simulink model "iddemo_engine"  (R2016a)
settings: Solver=ode45  StartTime=0.0  StopTime=200  MaxStep=0.01  RelTol=1e-3
model workspace (MAT data in the model file):
  Adist = -0.7
  N = 2000
  Tdist = 200
  Ts = 0.003
  p = [-7.82997288351e-05; 0.181210895977; -0.072497134344; 0.000486358314052; 0.0361674637937]
undefined symbols (not defined in the file or in its folder): magnitude
libraries: simulink x1, slident x1
settings Model: Creator=The MathWorks, Inc.  LastModifiedBy=The MathWorks, Inc.
settings DataIOCC: LimitDataPoints=on  SaveFormat=Array
settings DebuggingCC: SolverPrmCheckMsg=warning
settings HardwareCC: ProdBitPerPointer=32  ProdLargestAtomicFloat=None  ProdIntDivRoundTo=Undefined  ProdEndianess=Unspecified  ProdWordSize=32  ProdHWDeviceType=32-bit Generic
settings ModelReferenceCC: PropagateSignalLabelsOutOfModel=off
settings SFSimCC: SimGenImportedTypeDefs=on
settings ConfigComp: CovModelRefEnable=Off  CovSFcnEnable=off

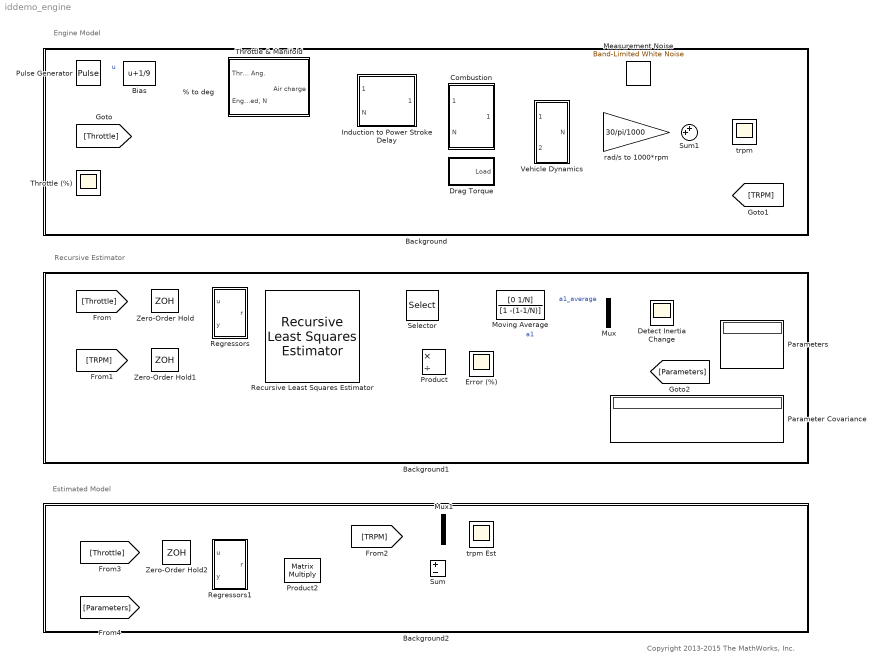
== system iddemo_engine ==
  note: Copyright 2013-2015 The MathWorks, Inc.
  note: Engine Model
  note: Recursive Estimator
  note: Estimated Model
  "% to deg " : Gain  Gain=90  SaturateOnIntegerOverflow=on  OutDataTypeStr=Inherit: Same as input  ParamDataTypeStr=Inherit: Same as input
  Background : Subsystem
      mask Display: disp('')
  Background1 : Subsystem
      mask Display: disp('')
  Background2 : Subsystem
      mask Display: disp('')
  Bias : Bias  Bias=1/9
  Combustion : Subsystem
      settings: RTWMemSecFuncInitTerm=Default  RTWMemSecFuncExecute=Default  RTWMemSecDataConstants=Default  RTWMemSecDataInternal=Default  RTWMemSecDataParameters=Default
  Detect Inertia Change : Scope
  Drag Torque : Subsystem
      settings: RTWMemSecFuncInitTerm=Default  RTWMemSecFuncExecute=Default  RTWMemSecDataConstants=Default  RTWMemSecDataInternal=Default  RTWMemSecDataParameters=Default
  Error (%) : Scope
  Induction to Power Stroke Delay : Subsystem
      settings: RTWMemSecFuncInitTerm=Default  RTWMemSecFuncExecute=Default  RTWMemSecDataConstants=Default  RTWMemSecDataInternal=Default  RTWMemSecDataParameters=Default
  Measurement Noise : simulink/Sources/Band-Limited White Noise  Cov=1e-5  Ts=Ts  seed=[23341]
  Moving Average : DiscreteFilter  Numerator=[0 1/N]  Denominator=[1 -(1-1/N)]
  Mux : Mux  Inputs=2
  Mux1 : Mux  Inputs=2
  Parameter Covariance : Display
  Parameters : Display
  Product : Product  Inputs=*/
  Product2 : Product  Multiplication=Matrix(*)
  Pulse Generator : DiscretePulseGenerator  PulseType=Time based  Amplitude=7/9  Period=20  PulseWidth=50
  Recursive Least Squares Estimator : slident/Estimators/Recursive Least Squares Estimator  InitialEstimateSource=None  InitialParameterData=3  P0=1  EstimationMethod=Forgetting Factor  AdaptationParameter=1-2e-4  NormalizationBias=eps  OutputError=on  OutputP=on  AddEnablePort=off  Ts=Ts
  Regressors : Subsystem
  Regressors1 : Subsystem
  Selector : Selector  InputPortWidth=3  IndexOptions=Index vector (dialog)  Indices=1  OutputSizes=1
  Sum : Sum  Inputs=+-
  Sum1 : Sum  Inputs=++|
  Throttle & Manifold : Subsystem
      settings: RTWMemSecFuncInitTerm=Default  RTWMemSecFuncExecute=Default  RTWMemSecDataConstants=Default  RTWMemSecDataInternal=Default  RTWMemSecDataParameters=Default
  Throttle (%) : Scope
  Vehicle Dynamics : Subsystem
      settings: RTWMemSecFuncInitTerm=Default  RTWMemSecFuncExecute=Default  RTWMemSecDataConstants=Default  RTWMemSecDataInternal=Default  RTWMemSecDataParameters=Default
  Zero-Order Hold : ZeroOrderHold  SampleTime=Ts
  Zero-Order Hold1 : ZeroOrderHold  SampleTime=Ts
  Zero-Order Hold2 : ZeroOrderHold  SampleTime=Ts
  rad/s to 1000*rpm : Gain  Gain=30/pi/1000  SaturateOnIntegerOverflow=on  OutDataTypeStr=Inherit: Same as input  ParamDataTypeStr=Inherit: Same as input
  trpm : Scope
  trpm Est : Scope  NumInputPorts=2
  wires:
  Throttle & Manifold/1(Air charge) -> Induction to Power Stroke Delay/1(Air charge)
  Vehicle Dynamics/1(N) -> Combustion/2(N), Induction to Power Stroke Delay/2(N), Throttle & Manifold/2("Engine Speed, N"), rad/s to 1000*rpm/1
  Combustion/1(Torque) -> Vehicle Dynamics/1(Teng)
  Drag Torque/1(Load) -> Vehicle Dynamics/2(Tload)
  Induction to Power Stroke Delay/1(Air Charge) -> Combustion/1(Air Charge)
  Pulse Generator/1 -> Bias/1  "u"
  Bias/1 -> Throttle (%)/1, [Throttle], "% to deg "/1
  Regressors/1(r) -> Recursive Least Squares Estimator/1
  Recursive Least Squares Estimator/1 -> Selector/1, [Parameters], Parameters/1
  Recursive Least Squares Estimator/2 -> Product/1
  Product/1 -> Error (%)/1
  [TRPM] -> Zero-Order Hold1/1
  Recursive Least Squares Estimator/3 -> Parameter Covariance/1
  Selector/1 -> Mux/2, Moving Average/1  "a1"
  [Throttle] -> Zero-Order Hold/1
  Moving Average/1 -> Mux/1  "a1_average"
  Mux/1 -> Detect Inertia Change/1
  Sum/1 -> trpm Est/2
  Regressors1/1(r) -> Product2/1
  [Throttle] -> Zero-Order Hold2/1
  [TRPM] -> Sum/1, Mux1/2
  Mux1/1 -> trpm Est/1
  Sum1/1 -> [TRPM], trpm/1
  rad/s to 1000*rpm/1 -> Sum1/2
  Measurement Noise/1 -> Sum1/1
  Zero-Order Hold/1 -> Regressors/1(u)
  Zero-Order Hold1/1 -> Recursive Least Squares Estimator/2, Regressors/2(y), Product/2
  Zero-Order Hold2/1 -> Regressors1/1(u)
  Product2/1 -> Sum/2, Regressors1/2(y), Mux1/1
  [Parameters] -> Product2/2
  "% to deg "/1 -> Throttle & Manifold/1(Throttle Ang.)

== system iddemo_engine/Background ==

== system iddemo_engine/Background1 ==

== system iddemo_engine/Background2 ==

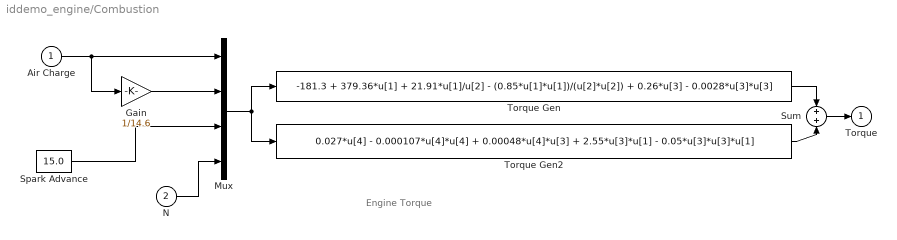
== system iddemo_engine/Combustion ==
  note: Engine Torque
  Air Charge : Inport
  N : Inport  Port=2
  Gain : Gain  Gain=1/14.6
  Mux : Mux
  Spark Advance : Constant  Value=15.0
  Sum : Sum  SaturateOnIntegerOverflow=on  InputSameDT=on  OutDataTypeStr=Inherit: Same as first input
  Torque Gen : Fcn  Expr=-181.3 + 379.36*u[1] + 21.91*u[1]/u[2] - (0.85*u[1]*u[1])/(u[2]*u[2]) + 0.26*u[3] - 0.0028*u[3]*u[3]
  Torque Gen2 : Fcn  Expr=0.027*u[4] - 0.000107*u[4]*u[4] + 0.00048*u[4]*u[3] + 2.55*u[3]*u[1] - 0.05*u[3]*u[3]*u[1]
  Torque : Outport  InitialOutput=0
  wires:
  Spark Advance/1 -> Mux/3
  N/1 -> Mux/4
  Air Charge/1 -> Gain/1, Mux/1
  Mux/1 -> Torque Gen/1, Torque Gen2/1
  Torque Gen2/1 -> Sum/2
  Torque Gen/1 -> Sum/1
  Sum/1 -> Torque/1
  Gain/1 -> Mux/2

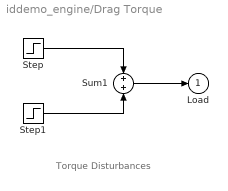
== system iddemo_engine/Drag Torque ==
  note: Torque Disturbances
  Step : Step  Time=45  After=0  SampleTime=0
  Step1 : Step  Time=45  After=0  SampleTime=0
  Sum1 : Sum  SaturateOnIntegerOverflow=on  InputSameDT=on  OutDataTypeStr=Inherit: Same as first input
  Load : Outport  InitialOutput=0
  wires:
  Step1/1 -> Sum1/2
  Step/1 -> Sum1/1
  Sum1/1 -> Load/1

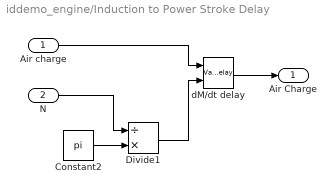
== system iddemo_engine/Induction to Power Stroke Delay ==
  Air charge : Inport
  N : Inport  Port=2
  Constant2 : Constant  Value=pi
  Divide1 : Product  Inputs=/*
  dM/dt delay : VariableTransportDelay  MaximumDelay=10  InitialOutput=0.152231307101552  MaximumPoints=5120  TransDelayFeedthrough=on  PadeOrder=2
  Air Charge : Outport
  wires:
  dM/dt delay/1 -> Air Charge/1
  Constant2/1 -> Divide1/2
  N/1 -> Divide1/1
  Divide1/1 -> dM/dt delay/2
  Air charge/1 -> dM/dt delay/1

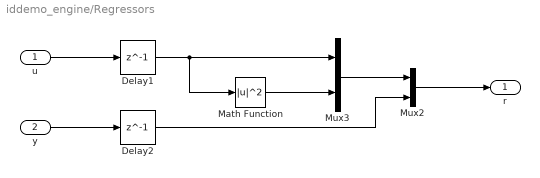
== system iddemo_engine/Regressors ==
  u : Inport
  y : Inport  Port=2
  Delay1 : Delay  DelayLength=1  InitialCondition=1  SampleTime=Ts
  Delay2 : Delay  DelayLength=1  InitialCondition=2  SampleTime=Ts
  Math Function : Math  Operator=magnitude^2  SaturateOnIntegerOverflow=on
  Mux2 : Mux  Inputs=2
  Mux3 : Mux  Inputs=2
  r : Outport
  wires:
  u/1 -> Delay1/1
  Mux2/1 -> r/1
  Delay1/1 -> Math Function/1, Mux3/1
  y/1 -> Delay2/1
  Mux3/1 -> Mux2/1
  Delay2/1 -> Mux2/2
  Math Function/1 -> Mux3/2

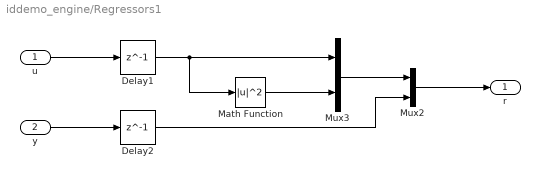
== system iddemo_engine/Regressors1 ==
  u : Inport
  y : Inport  Port=2
  Delay1 : Delay  DelayLength=1  InitialCondition=1  SampleTime=Ts
  Delay2 : Delay  DelayLength=1  InitialCondition=2  SampleTime=Ts
  Math Function : Math  Operator=magnitude^2  SaturateOnIntegerOverflow=on
  Mux2 : Mux  Inputs=2
  Mux3 : Mux  Inputs=2
  r : Outport
  wires:
  u/1 -> Delay1/1
  Mux2/1 -> r/1
  Delay1/1 -> Math Function/1, Mux3/1
  y/1 -> Delay2/1
  Mux3/1 -> Mux2/1
  Delay2/1 -> Mux2/2
  Math Function/1 -> Mux3/2

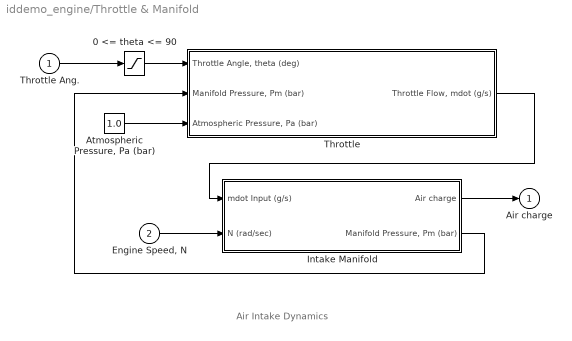
== system iddemo_engine/Throttle & Manifold ==
  note: Air Intake Dynamics
  Throttle Ang. : Inport
  "Engine Speed, N" : Inport  Port=2
  0 <= theta <= 90 : Saturate  UpperLimit=90  LowerLimit=0
  "Atmospheric Pressure, Pa (bar)" : Constant  Value=1.0
  Intake Manifold : Subsystem
      settings: RTWMemSecFuncInitTerm=Default  RTWMemSecFuncExecute=Default  RTWMemSecDataConstants=Default  RTWMemSecDataInternal=Default  RTWMemSecDataParameters=Default
  Throttle : Subsystem
      settings: RTWMemSecFuncInitTerm=Default  RTWMemSecFuncExecute=Default  RTWMemSecDataConstants=Default  RTWMemSecDataInternal=Default  RTWMemSecDataParameters=Default
  Air charge : Outport  InitialOutput=0
  wires:
  Intake Manifold/1(Air charge) -> Air charge/1
  Intake Manifold/2("Manifold Pressure, Pm (bar)") -> Throttle/2("Manifold Pressure, Pm (bar)")
  "Engine Speed, N"/1 -> Intake Manifold/2(N (rad/sec))
  Throttle/1("Throttle Flow, mdot (g/s)") -> Intake Manifold/1(mdot Input (g/s))
  Throttle Ang./1 -> 0 <= theta <= 90/1
  0 <= theta <= 90/1 -> Throttle/1("Throttle Angle, theta (deg)")
  "Atmospheric Pressure, Pa (bar)"/1 -> Throttle/3("Atmospheric Pressure, Pa (bar) ")

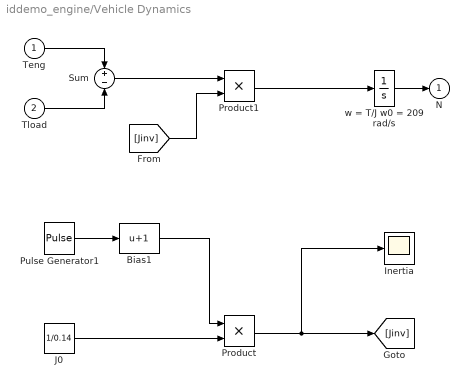
== system iddemo_engine/Vehicle Dynamics ==
  Teng : Inport
  Tload : Inport  Port=2
  Bias1 : Bias  Bias=1
  Inertia : Scope
  J0 : Constant  Value=1/0.14
  Product : Product
  Product1 : Product
  Pulse Generator1 : DiscretePulseGenerator  PulseType=Time based  Amplitude=Adist  Period=Tdist  PulseWidth=50  PhaseDelay=Tdist/2
  Sum : Sum  Inputs=+-  SaturateOnIntegerOverflow=on  InputSameDT=on  OutDataTypeStr=Inherit: Same as first input
  w = T/J w0 = 209 rad/s : Integrator  InitialCondition=209.4395102393211
  N : Outport  InitialOutput=0
  wires:
  Product1/1 -> w = T/J w0 = 209 rad/s/1
  w = T/J w0 = 209 rad/s/1 -> N/1
  Sum/1 -> Product1/1
  Teng/1 -> Sum/1
  Tload/1 -> Sum/2
  Pulse Generator1/1 -> Bias1/1
  J0/1 -> Product/2
  Bias1/1 -> Product/1
  Product/1 -> Inertia/1, [Jinv]
  [Jinv] -> Product1/2

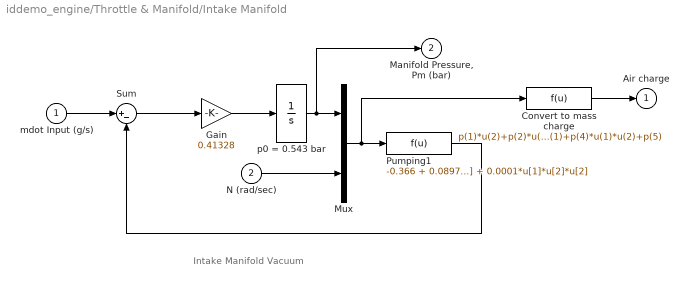
== system iddemo_engine/Throttle & Manifold/Intake Manifold ==
  note: Intake Manifold Vacuum
  mdot Input (g/s) : Inport
  N (rad/sec) : Inport  Port=2
  Convert to mass charge : Fcn  Expr=p(1)*u(2)+p(2)*u(1)+p(3)*u(1)*u(1)+p(4)*u(1)*u(2)+p(5)
  Gain : Gain  Gain=0.41328
  Mux : Mux  Inputs=2
  Pumping1 : Fcn  Expr=-0.366 + 0.08979*u[1]*u[2] - 0.0337*u[2]*u[1]*u[1] + 0.0001*u[1]*u[2]*u[2]
  Sum : Sum  Inputs=|+-  SaturateOnIntegerOverflow=on  InputSameDT=on  OutDataTypeStr=Inherit: Same as first input
  p0 = 0.543 bar : Integrator  InitialCondition=0.543634736225556
  Air charge : Outport  InitialOutput=0
  "Manifold Pressure, Pm (bar)" : Outport  Port=2  InitialOutput=0
  wires:
  Pumping1/1 -> Sum/2
  Sum/1 -> Gain/1
  p0 = 0.543 bar/1 -> "Manifold Pressure, Pm (bar)"/1, Mux/1
  Mux/1 -> Pumping1/1, Convert to mass charge/1
  N (rad/sec)/1 -> Mux/2
  Gain/1 -> p0 = 0.543 bar/1
  mdot Input (g/s)/1 -> Sum/1
  Convert to mass charge/1 -> Air charge/1

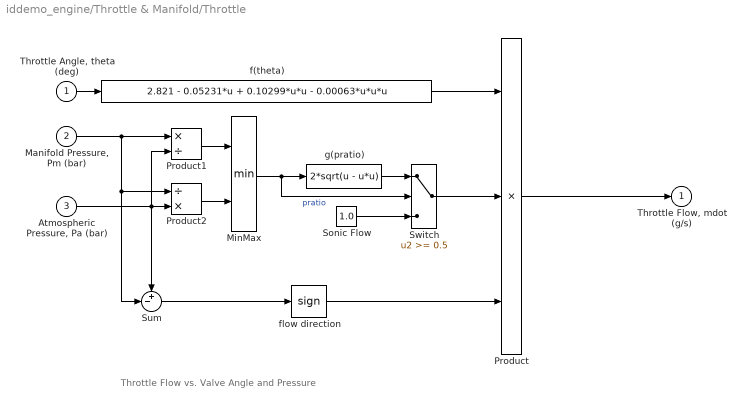
== system iddemo_engine/Throttle & Manifold/Throttle ==
  note: Throttle Flow vs. Valve Angle and Pressure
  "Throttle Angle, theta (deg)" : Inport
  "Manifold Pressure, Pm (bar)" : Inport  Port=2
  "Atmospheric Pressure, Pa (bar) " : Inport  Port=3
  MinMax : MinMax  Inputs=2  SaturateOnIntegerOverflow=on  InputSameDT=on
  Product : Product  Inputs=3  SaturateOnIntegerOverflow=on  RndMeth=Zero  InputSameDT=on  OutDataTypeStr=Inherit: Same as first input
  Product1 : Product  Inputs=*/  SaturateOnIntegerOverflow=on  RndMeth=Zero  InputSameDT=on  OutDataTypeStr=Inherit: Same as first input
  Product2 : Product  Inputs=/*  SaturateOnIntegerOverflow=on  RndMeth=Zero  InputSameDT=on  OutDataTypeStr=Inherit: Same as first input
  "Sonic Flow " : Constant  Value=1.0
  Sum : Sum  Inputs=+-|  SaturateOnIntegerOverflow=on  InputSameDT=on  OutDataTypeStr=Inherit: Same as first input
  Switch : Switch  Threshold=0.5  SaturateOnIntegerOverflow=on  InputSameDT=on
  f(theta) : Fcn  Expr=2.821 - 0.05231*u + 0.10299*u*u - 0.00063*u*u*u
  flow direction : Signum
  g(pratio) : Fcn  Expr=2*sqrt(u - u*u)
  "Throttle Flow, mdot (g/s)" : Outport  InitialOutput=0
  wires:
  "Throttle Angle, theta (deg)"/1 -> f(theta)/1
  MinMax/1 -> g(pratio)/1, Switch/2  "pratio"
  Sum/1 -> flow direction/1
  flow direction/1 -> Product/3
  "Sonic Flow "/1 -> Switch/3
  g(pratio)/1 -> Switch/1
  "Atmospheric Pressure, Pa (bar) "/1 -> Product2/2, Sum/1, Product1/2
  Product1/1 -> MinMax/1
  Product2/1 -> MinMax/2
  "Manifold Pressure, Pm (bar)"/1 -> Product1/1, Product2/1, Sum/2
  f(theta)/1 -> Product/1
  Switch/1 -> Product/2
  Product/1 -> "Throttle Flow, mdot (g/s)"/1
